simulink model "IMU_int"  (R2023b)
settings: Solver=ode3  StartTime=0.0  StopTime=10  FixedStep=clock.sampleTime.value  RelTol=1e-3
undefined symbols (not defined in the file or in its folder): x0
libraries: nav_lib x3, sharedtransform x2, dyn_lib x1
settings Model: DataDictionary=SimulationDict.sldd  EnableAccessToBaseWorkspace=off  Creator=brent  LastModifiedBy=brent

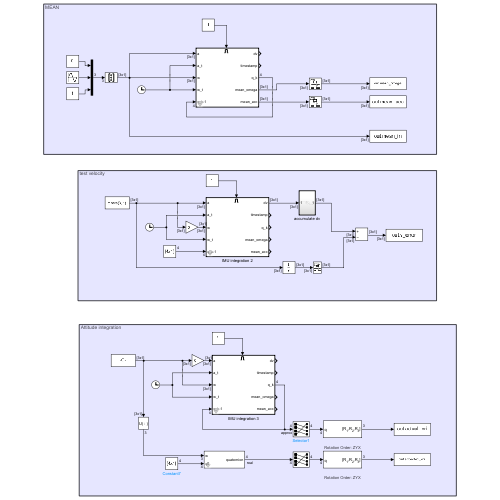
[thumbnail: Simulink's stored preview of the top-level diagram]
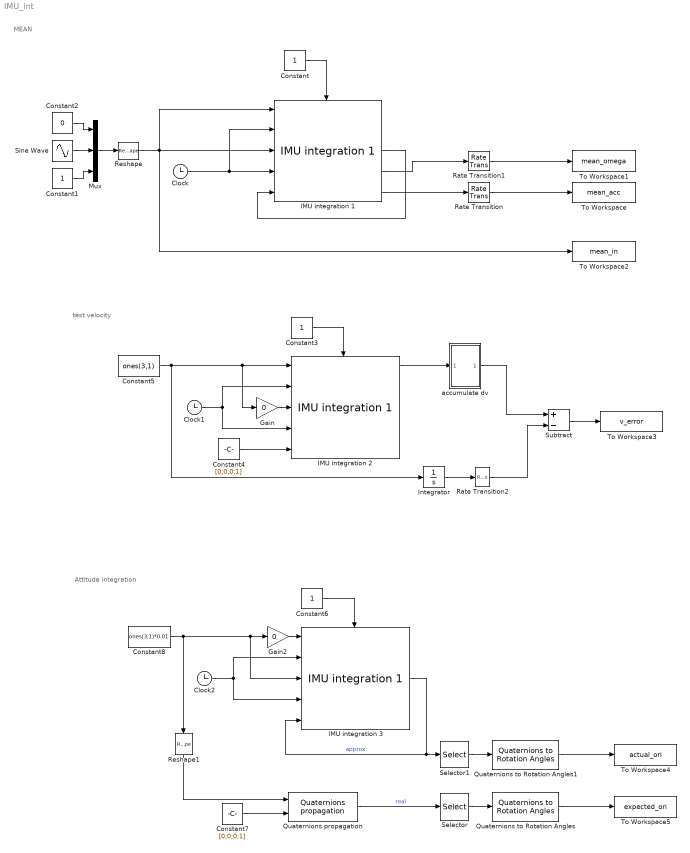
== system IMU_int ==
  note: Attitude integration
  note: test velocity
  note: MEAN
  Clock : Clock
  Clock1 : Clock
  Clock2 : Clock
  Constant{,1,3,6} (4 alike) : Constant
  Constant2 : Constant  Value=0
  Constant4 : Constant  Value=[0;0;0;1]
  Constant5 : Constant  Value=ones(3,1)  VectorParams1D=off
  Constant7 : Constant  Value=[0;0;0;1]
  Constant8 : Constant  Value=ones(3,1)*0.01  VectorParams1D=off
  Gain : Gain  Gain=0
  Gain2 : Gain  Gain=0
  IMU integration 1 : nav_lib/IMU integration 1  q0=x0.value(7:10)  HF=Propagation.hf.value  LF=Propagation.lf.value
      settings: SourceProductName=Navigation library
  IMU integration 2 : nav_lib/IMU integration 1  q0=[0;0;0;1]  HF=Propagation.hf.value  LF=Propagation.lf.value
      settings: SourceProductName=Navigation library
  IMU integration 3 : nav_lib/IMU integration 1  q0=[0;0;0;1]  HF=Propagation.hf.value  LF=Propagation.lf.value
      settings: SourceProductName=Navigation library
  Integrator : Integrator
  Mux : Mux  Inputs=3
  Quaternions propagation : dyn_lib/Quaternions propagation
      settings: SourceProductName=Dynamics library
  Quaternions to Rotation Angles : sharedtransform/Quaternions to Rotation Angles  rotationOrder=ZYX  aMode=aMode
  Quaternions to Rotation Angles1 : sharedtransform/Quaternions to Rotation Angles  rotationOrder=ZYX  aMode=aMode
  Rate Transition : RateTransition  OutPortSampleTime=0.2
  Rate Transition1 : RateTransition  OutPortSampleTime=0.2
  Rate Transition2 : RateTransition  OutPortSampleTime=0.2
  Reshape : Reshape  OutputDimensionality=Column vector (2-D)
  Reshape1 : Reshape
  Selector : Selector  InputPortWidth=4  IndexOptions=Index vector (dialog)  Indices=[4 1 2 3]  OutputSizes=1
  Selector1 : Selector  InputPortWidth=4  IndexOptions=Index vector (dialog)  Indices=[4 1 2 3]  OutputSizes=1
  Sine Wave : Sin  SampleTime=0
  Subtract : Sum  Inputs=+-
  To Workspace : ToWorkspace  VariableName=mean_acc  SampleTime=-1
  To Workspace1 : ToWorkspace  VariableName=mean_omega  SampleTime=-1
  To Workspace2 : ToWorkspace  VariableName=mean_in  SampleTime=-1
  To Workspace3 : ToWorkspace  VariableName=v_error  SampleTime=-1
  To Workspace4 : ToWorkspace  VariableName=actual_ori  SampleTime=-1
  To Workspace5 : ToWorkspace  VariableName=expected_ori  SampleTime=-1
  accumulate dv : Subsystem  TreatAsAtomicUnit=on  SystemSampleTime=0.2
  wires:
  Constant/1 -> IMU integration 1/Enable
  IMU integration 1/3 -> IMU integration 1/5
  Clock/1 -> IMU integration 1/2, IMU integration 1/4
  Mux/1 -> Reshape/1
  Constant1/1 -> Mux/3
  Sine Wave/1 -> Mux/2
  Constant2/1 -> Mux/1
  Rate Transition/1 -> To Workspace/1
  Rate Transition1/1 -> To Workspace1/1
  Reshape/1 -> To Workspace2/1, IMU integration 1/1, IMU integration 1/3
  IMU integration 1/5 -> Rate Transition/1
  IMU integration 1/4 -> Rate Transition1/1
  Constant3/1 -> IMU integration 2/Enable
  Constant4/1 -> IMU integration 2/5
  Clock1/1 -> IMU integration 2/2, IMU integration 2/4
  Constant5/1 -> IMU integration 2/1, Gain/1, Integrator/1
  Gain/1 -> IMU integration 2/3
  Integrator/1 -> Rate Transition2/1
  Subtract/1 -> To Workspace3/1
  IMU integration 2/1 -> accumulate dv/1(In1)
  accumulate dv/1(Out1) -> Subtract/1
  Rate Transition2/1 -> Subtract/2
  Constant6/1 -> IMU integration 3/Enable
  Constant8/1 -> Reshape1/1, IMU integration 3/3, Gain2/1
  Clock2/1 -> IMU integration 3/2, IMU integration 3/4
  Gain2/1 -> IMU integration 3/1
  IMU integration 3/3 -> Selector1/1, IMU integration 3/5  "approx"
  Constant7/1 -> Quaternions propagation/2
  Reshape1/1 -> Quaternions propagation/1
  Quaternions propagation/1 -> Selector/1  "real"
  Selector/1 -> Quaternions to Rotation Angles/1
  Selector1/1 -> Quaternions to Rotation Angles1/1
  Quaternions to Rotation Angles1/1 -> To Workspace4/1
  Quaternions to Rotation Angles/1 -> To Workspace5/1

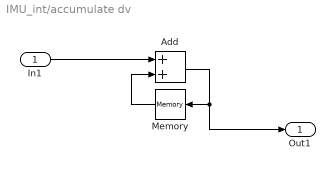
== system IMU_int/accumulate dv ==
  In1 : Inport
  Add : Sum
  Memory : Memory  InheritSampleTime=on
  Out1 : Outport
  wires:
  Add/1 -> Out1/1, Memory/1
  Memory/1 -> Add/2
  In1/1 -> Add/1
